simulink model "LQG_to_ply_with_mac"  (R2019b)
settings: Solver=FixedStepAuto  StartTime=0.0  StopTime=100  FixedStep=.0001  RelTol=1e-3
values from neighbouring files (symbols this model uses):
  Fes = F-L*H    [KF3_Script.m]    (also in KF_Script.m; LQG_Script.m)
  K = dlqr(F(1:2,1:2),G(1:2),[1 0;0 .1],0.01)    [LQG_Script.m]
  Kt = 0.071    [KF3_Script.m]    (also in KF_Script.m; LQG_Script.m)
  L = (dlqr(F',H',Q,R))'    [KF3_Script.m]    (also in KF_Script.m; LQG_Script.m)
undefined symbols (not defined in the file or in its folder): G
libraries: simulink x2
settings Model: Creator=oboe  LastModifiedBy=oboe
settings DataIOCC: LimitDataPoints=on  SaveFormat=Array  ReturnWorkspaceOutputs=off
settings OptimizationCC: LifeSpan=inf
settings DebuggingCC: SolverPrmCheckMsg=warning  SFUnexpectedBacktrackingDiag=warning  SFNoUnconditionalDefaultTransitionDiag=warning  SFExecutionAtInitializationDiag=none  ArithmeticOperatorsInVariantConditions=warning
settings HardwareCC: ProdBitPerPointer=32  ProdBitPerSizeT=32  ProdBitPerPtrDiffT=32  ProdLargestAtomicFloat=None  ProdIntDivRoundTo=Undefined  ProdEndianess=Unspecified  ProdWordSize=32  ProdHWDeviceType=32-bit Generic
settings ModelReferenceCC: PropagateSignalLabelsOutOfModel=off
settings SFSimCC: SimUseLocalCustomCode=off  CustomCodeUndefinedFunction=UseInterfaceOnly
settings RTWCC: RTWUseLocalCustomCode=off
settings CodeAppCC: StateflowObjectComments=on
settings GRTTargetCC: TargetLangStandard=C89/C90 (ANSI)  GeneratePreprocessorConditionals=Disable all
settings ConfigComp: CovMetricSettings=dw  CovHtmlReporting=on  CovSaveCumulativeToWorkspaceVar=on  CovSaveSingleToWorkspaceVar=on  CovExternalEMLEnable=off  CovSFcnEnable=off

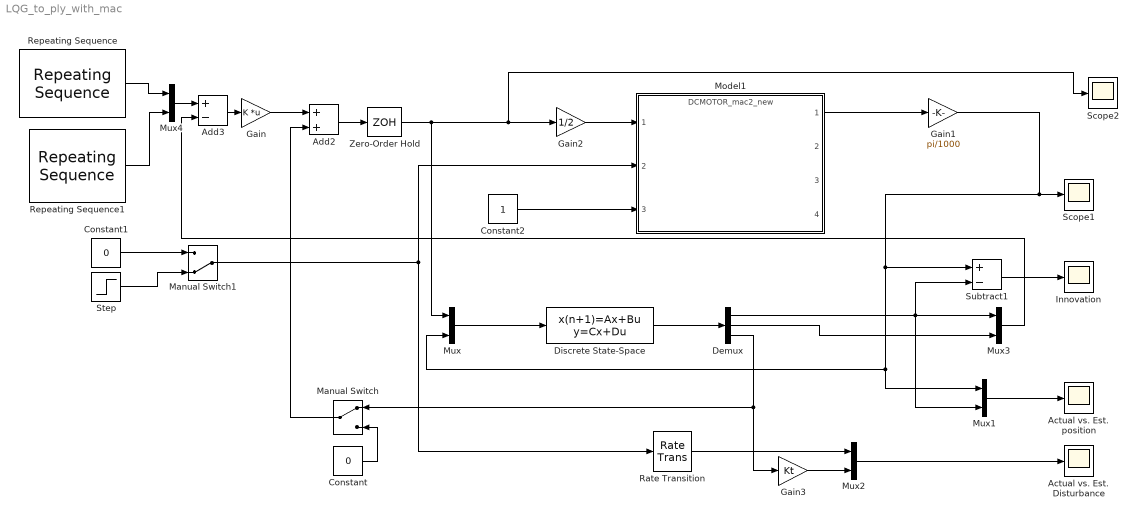
== system LQG_to_ply_with_mac ==
  Actual vs. Est. Disturbance : Scope
  Actual vs. Est. position : Scope
  Add2 : Sum
  Add3 : Sum  Inputs=+-
  Constant : Constant  Value=0
  Constant1 : Constant  Value=0
  Constant2 : Constant
  Demux : Demux  Outputs=3
  Discrete State-Space : DiscreteStateSpace  A=Fes  B=[G L]  C=eye(3)  D=zeros(3,2)  SampleTime=.001
  Gain : Gain  Gain=K  Multiplication=Matrix(K*u)
  Gain1 : Gain  Gain=pi/1000
  Gain2 : Gain  Gain=1/2
  Gain3 : Gain  Gain=Kt
  Innovation : Scope
  Manual Switch : ManualSwitch
  Manual Switch1 : ManualSwitch  CurrentSetting=0
  Model1 : ModelReference  ModelNameDialog=DCMOTOR_mac2_new.slxp  ModelReferenceVersion=1.21  CopyOfModelProtected=on
  Mux{,1..4} (5 alike) : Mux  Inputs=2
  Rate Transition : RateTransition
  Repeating Sequence : simulink/Sources/Repeating Sequence  rep_seq_t=[0 1 2 3 4]  rep_seq_y=[0 0 1 1 0]
  Repeating Sequence1 : simulink/Sources/Repeating Sequence  rep_seq_t=[0 1-0.001 1 2-0.001 2 3-0.001 3 4-0.001 4]  rep_seq_y=[0 0 1 1 0 0 -1 -1 0]
  Scope1 : Scope
  Scope2 : Scope
  Step : Step  After=.1  SampleTime=0
  Subtract1 : Sum  Inputs=+-
  Zero-Order Hold : ZeroOrderHold  SampleTime=0.001
  wires:
  Mux/1 -> Discrete State-Space/1
  Discrete State-Space/1 -> Demux/1
  Demux/1 -> Mux3/1, Mux1/2, Subtract1/2
  Mux1/1 -> Actual vs. Est. position/1
  Subtract1/1 -> Innovation/1
  Gain1/1 -> Mux/2, Mux1/1, Subtract1/1, Scope1/1
  Gain/1 -> Add2/1
  Add2/1 -> Zero-Order Hold/1
  Demux/3 -> Manual Switch/1, Gain3/1
  Mux2/1 -> Actual vs. Est. Disturbance/1
  Demux/2 -> Mux3/2
  Repeating Sequence/1 -> Mux4/1
  Repeating Sequence1/1 -> Mux4/2
  Mux4/1 -> Add3/1
  Mux3/1 -> Add3/2
  Add3/1 -> Gain/1
  Manual Switch/1 -> Add2/2
  Constant/1 -> Manual Switch/2
  Constant1/1 -> Manual Switch1/1
  Step/1 -> Manual Switch1/2
  Model1/1 -> Gain1/1
  Zero-Order Hold/1 -> Mux/1, Scope2/1, Gain2/1
  Gain2/1 -> Model1/1
  Manual Switch1/1 -> Rate Transition/1, Model1/2
  Gain3/1 -> Mux2/2
  Constant2/1 -> Model1/3
  Rate Transition/1 -> Mux2/1
